simulink model "three_phase_inverter"  (R2021a)
settings: Solver=ode23tb  StartTime=0.0  StopTime=0.5  MaxStep=1e-4  RelTol=1e-3
values from neighbouring files (symbols this model uses):
  Ac = 1    [Inverter_parameters.m]
  Ar = ma*Ac    (= 0.5)    [Inverter_parameters.m]
  Cf = 0.05*Cb    (= 1.42154514158e-05)    [LCL_design.m]
  fc1 = mf1*f    (= 1000)    [Inverter_parameters.m]
  fr = 2*pi*f    (= 314.159265359)    [Inverter_parameters.m]
  L = X/(2*pi*f)    (= 0.0999493042617)    [Inverter_parameters.m]
  L1 = Vdc/(6*Fsw*delta_Imax)    [LCL_design.m]
  L2 = 0.6*L1    [LCL_design.m]
  R = 100    [Inverter_parameters.m]
  Rf = 1/(3*Cf*wres)    [LCL_design.m]
  Vin = 780    [Inverter_parameters.m]
libraries: spsIGBTDiodeLib x6, spsRMSLib x6, spsThreePhaseSeriesRLCBranchLib x4, spsThreePhaseVIMeasurementLib x2, spsCurrentMeasurementLib x1, spsGroundLib x1, spsDCVoltageSourceLib x1, simulink x1, spspowerguiLib x1
settings Model: Creator=HossamAladdin  LastModifiedBy=HossamAladdin
settings DataIOCC: ReturnWorkspaceOutputs=off

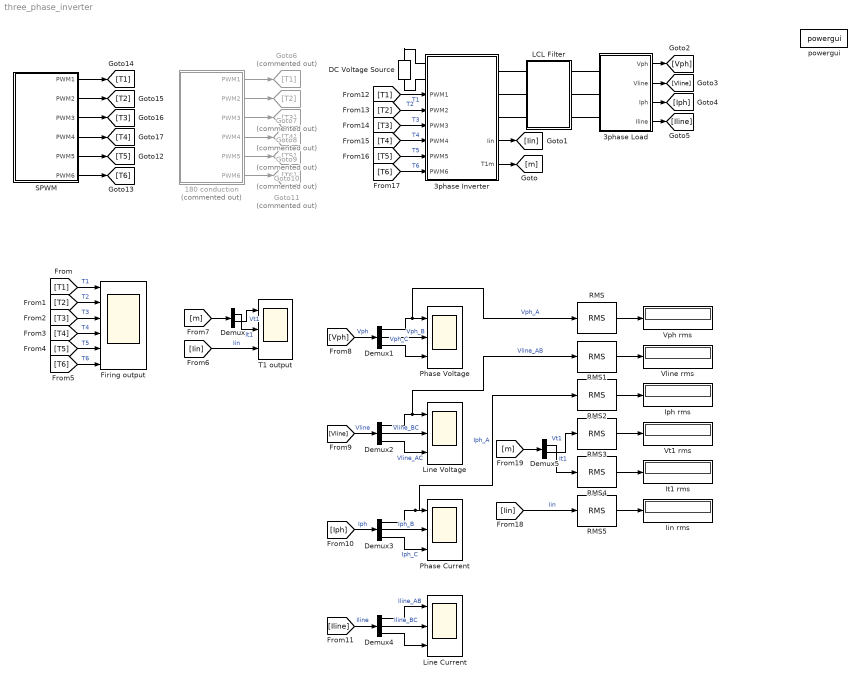
== system three_phase_inverter ==
  180 conduction : Subsystem  Commented=on
  3phase Inverter : Subsystem
      settings: PortSchema="{\"entries\":[{\"content\":{\"sides\":[{\"content\":{\"connectorIds\":[\"LConn1\",\"LConn2\",\"In1\",\"In2\",\"In3\",\"In4\",\"In5\",\"In6\"]},\"type\":\"ConnectorPlacement.EquallySpacedRectSide\",\"uuid\":\"d07aecf3-188f-425b-a441-0ff53fdce9b7\"},{\"content\":{\"connectorIds\":[\"RConn1\",\"RConn2\",\"RConn3\",\"Out1\",\"Out2\"],\"side\":\"RIGHT\"},\"type\":\"ConnectorPlacement.EquallySpacedRectSide\",\"uuid\":\"cba8ab7f-84b3-4f09-b5c1-8f8cbc780d5b\"},{\"content\":{\"connectorIds\":[],\"side\":\"TOP\"},\"type\":\"ConnectorPlacement.EquallySpacedRectSide\",\"uuid\":\"7fc08851-147a-460f-9c9e-af6a73bd199d\"}]},\"type\":\"ConnectorPlacement.EquallySpacedConnector\",\"uuid\":\"b80a74c3-b878-4e7f-834a-08d1a7e19c1c\"}],\"packageUris\":[\"http://schema.mathworks.com/mf0/Connector/R2020b\"],\"version\":\"1.0\"}"
  3phase Load : Subsystem
  DC Voltage Source : spsDCVoltageSourceLib/DC Voltage Source  Amplitude=Vin  Measurements=None
  Demux : Demux  Outputs=2
  Demux{1..4} (4 alike) : Demux  Outputs=3
  Demux5 : Demux  Outputs=2
  Firing output : Scope  NumInputPorts=6
  Goto10 : Goto  Commented=on  GotoTag=T5
  Goto11 : Goto  Commented=on  GotoTag=T6
  Goto6 : Goto  Commented=on  GotoTag=T1
  Goto7 : Goto  Commented=on  GotoTag=T2
  Goto8 : Goto  Commented=on  GotoTag=T3
  Goto9 : Goto  Commented=on  GotoTag=T4
  Iin rms : Display
  Iph rms : Display
  It1 rms : Display
  LCL Filter : Subsystem
  Line Current : Scope  NumInputPorts=3
  Line Voltage : Scope  NumInputPorts=3
  Phase Current : Scope  NumInputPorts=3
  Phase Voltage : Scope  NumInputPorts=3
  RMS{,1..5} (6 alike) : spsRMSLib/RMS  TrueRMS=on  Freq=50  RMSInit=0  Ts=0
  SPWM : Subsystem
  T1 output : Scope  NumInputPorts=3
  Vline rms : Display
  Vph rms : Display
  Vt1 rms : Display
  powergui : spspowerguiLib/powergui  Priority=1  SimulationMode=Discrete  SampleTime=1e-6  frequency=60  Iterations=50  frequencyindice=0  Pbase=100e6  ErrMax=1e-4  UnitsV=kV  UnitsW=MW  buscounter=0  FunctionMessages=off  echomessages=off  EnableUseOfTLC=off  CurrentSourceSwitches=off  DisableSnubberDevices=off  DisableRonSwitches=off  DisableVfSwitches=off  DisplayEquations=off  AutomaticDiscreteSolvers=off  SolverType=Tustin/Backward Euler (TBE)  Interpol=off  ExternalGateDelay=off  methode=off  Ts=100  x0status=blocks  SPID=on  SwTol=0  HookPort=off  NonlinearTolerance=1e-4  nMaxIteration=100  ContinueOnMaxIteration=off  RestoreLinks=warning  ResistiveCurrentMeasurement=off  Frange=[0:2:500]  Ylog=off  Xlog=on  ShowGrid=off  save=off  variable=ZData  structure=0  ZoomFFT=off  StartTime=0.0  cycles=1  DisplayStyle=1  fundamental=60  FreqAxis=off  MaxFrequency=1000  frequencyindicesteady=1  RmsSteady=1  display=off
  wires:
  180 conduction/6(PWM6) -> Goto11/1
  180 conduction/3(PWM3) -> Goto8/1
  180 conduction/1(PWM1) -> Goto6/1
  180 conduction/5(PWM5) -> Goto10/1
  180 conduction/2(PWM2) -> Goto7/1
  180 conduction/4(PWM4) -> Goto9/1
  3phase Inverter/2(T1m) -> [m]
  3phase Inverter/1(Iin) -> [Iin]
  [T1] -> Firing output/1  "T1"
  [T2] -> Firing output/2  "T2"
  [T3] -> Firing output/3  "T3"
  [T4] -> Firing output/4  "T4"
  [T5] -> Firing output/5  "T5"
  [T6] -> Firing output/6  "T6"
  [Iin] -> T1 output/3  "Iin"
  [m] -> Demux/1
  Demux/1 -> T1 output/2  "It1"
  Demux/2 -> T1 output/1  "Vt1"
  3phase Load/1(Vph) -> [Vph]
  3phase Load/2(Vline) -> [Vline]
  3phase Load/3(Iph) -> [Iph]
  3phase Load/4(Iline) -> [Iline]
  [Vph] -> Demux1/1  "Vph"
  [Vline] -> Demux2/1  "Vline"
  [Iph] -> Demux3/1  "Iph"
  [Iline] -> Demux4/1  "Iline"
  [T1] -> 3phase Inverter/1(PWM1)  "T1"
  [T6] -> 3phase Inverter/6(PWM6)  "T6"
  [T5] -> 3phase Inverter/5(PWM5)  "T5"
  [T4] -> 3phase Inverter/4(PWM4)  "T4"
  [T3] -> 3phase Inverter/3(PWM3)  "T3"
  [T2] -> 3phase Inverter/2(PWM2)  "T2"
  SPWM/4(PWM4) -> [T4]
  SPWM/2(PWM2) -> [T2]
  SPWM/5(PWM5) -> [T5]
  SPWM/1(PWM1) -> [T1]
  SPWM/3(PWM3) -> [T3]
  SPWM/6(PWM6) -> [T6]
  Demux1/1 -> RMS/1, Phase Voltage/1  "Vph_A"
  Demux1/2 -> Phase Voltage/2  "Vph_B"
  Demux1/3 -> Phase Voltage/3  "Vph_C"
  Demux2/1 -> RMS1/1, Line Voltage/1  "Vline_AB"
  Demux2/2 -> Line Voltage/2  "Vline_BC"
  Demux2/3 -> Line Voltage/3  "Vline_AC"
  Demux4/1 -> Line Current/1  "Iline_AB"
  Demux4/2 -> Line Current/2  "Iline_BC"
  Demux4/3 -> Line Current/3
  Demux3/1 -> RMS2/1, Phase Current/1  "Iph_A"
  Demux3/2 -> Phase Current/2  "Iph_B"
  Demux3/3 -> Phase Current/3  "Iph_C"
  RMS2/1 -> Iph rms/1
  RMS1/1 -> Vline rms/1
  RMS/1 -> Vph rms/1
  RMS4/1 -> It1 rms/1
  RMS3/1 -> Vt1 rms/1
  Demux5/2 -> RMS3/1  "Vt1"
  Demux5/1 -> RMS4/1  "It1"
  [m] -> Demux5/1
  [Iin] -> RMS5/1  "Iin"
  RMS5/1 -> Iin rms/1
  connections:
  DC Voltage Source/RConn1 -- 3phase Inverter/LConn1
  DC Voltage Source/LConn1 -- 3phase Inverter/LConn2
  LCL Filter/RConn1 -- 3phase Load/LConn1
  LCL Filter/RConn2 -- 3phase Load/LConn2
  LCL Filter/RConn3 -- 3phase Load/LConn3
  LCL Filter/LConn3 -- 3phase Inverter/RConn3
  LCL Filter/LConn1 -- 3phase Inverter/RConn1
  LCL Filter/LConn2 -- 3phase Inverter/RConn2

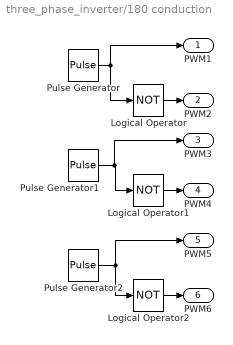
== system three_phase_inverter/180 conduction ==
  Logical Operator : Logic  Operator=NOT  AllPortsSameDT=off  OutDataTypeStr=boolean
  Logical Operator1 : Logic  Operator=NOT  AllPortsSameDT=off  OutDataTypeStr=boolean
  Logical Operator2 : Logic  Operator=NOT  AllPortsSameDT=off  OutDataTypeStr=boolean
  Pulse Generator : DiscretePulseGenerator  PulseType=Time based  Period=t  PulseWidth=50
  Pulse Generator1 : DiscretePulseGenerator  PulseType=Time based  Period=t  PulseWidth=50  PhaseDelay=(120*t)/360
  Pulse Generator2 : DiscretePulseGenerator  PulseType=Time based  Period=t  PulseWidth=50  PhaseDelay=(240*t)/360
  PWM1 : Outport
  PWM2 : Outport  Port=2
  PWM3 : Outport  Port=3
  PWM4 : Outport  Port=4
  PWM5 : Outport  Port=5
  PWM6 : Outport  Port=6
  wires:
  Logical Operator2/1 -> PWM6/1
  Logical Operator1/1 -> PWM4/1
  Pulse Generator/1 -> PWM1/1, Logical Operator/1
  Pulse Generator2/1 -> PWM5/1, Logical Operator2/1
  Pulse Generator1/1 -> PWM3/1, Logical Operator1/1
  Logical Operator/1 -> PWM2/1

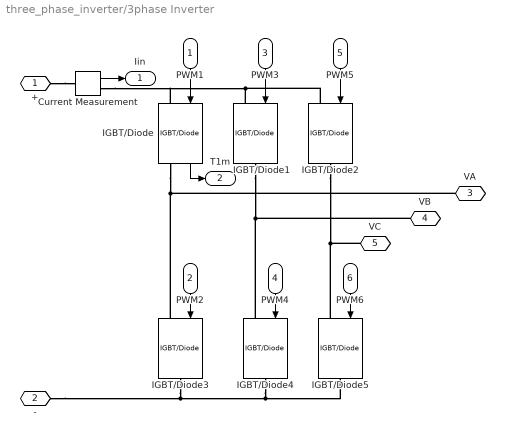
== system three_phase_inverter/3phase Inverter ==
  PWM1 : Inport
  PWM2 : Inport  Port=2
  PWM3 : Inport  Port=3
  PWM4 : Inport  Port=4
  PWM5 : Inport  Port=5
  PWM6 : Inport  Port=6
  Current Measurement : spsCurrentMeasurementLib/Current Measurement  PhasorSimulation=off  OutputType=Complex  PSBequivalent=0
  IGBT/Diode : spsIGBTDiodeLib/IGBT//Diode  Ron=1e-3  Rs=1e5  Cs=inf  Measurements=on
  IGBT/Diode{1..5} (5 alike) : spsIGBTDiodeLib/IGBT//Diode  Ron=1e-3  Rs=1e5  Cs=inf  Measurements=off
  + : PMIOPort  Side=Left
  - : PMIOPort  Port=2  Side=Left
  VA : PMIOPort  Port=3  Side=Right
  VB : PMIOPort  Port=4  Side=Right
  VC : PMIOPort  Port=5  Side=Right
  Iin : Outport
  T1m : Outport  Port=2
  wires:
  PWM1/1 -> IGBT/Diode/1
  PWM3/1 -> IGBT/Diode1/1
  PWM6/1 -> IGBT/Diode5/1
  PWM4/1 -> IGBT/Diode4/1
  PWM5/1 -> IGBT/Diode2/1
  PWM2/1 -> IGBT/Diode3/1
  IGBT/Diode/1 -> T1m/1
  Current Measurement/1 -> Iin/1
  connections:
  IGBT/Diode3/RConn1 -- IGBT/Diode5/RConn1 -- IGBT/Diode4/RConn1 -- -/RConn1
  IGBT/Diode2/LConn1 -- Current Measurement/RConn1 -- IGBT/Diode/LConn1 -- IGBT/Diode1/LConn1
  IGBT/Diode1/RConn1 -- VB/RConn1 -- IGBT/Diode4/LConn1
  IGBT/Diode2/RConn1 -- VC/RConn1 -- IGBT/Diode5/LConn1
  VA/RConn1 -- IGBT/Diode/RConn1 -- IGBT/Diode3/LConn1
  +/RConn1 -- Current Measurement/LConn1

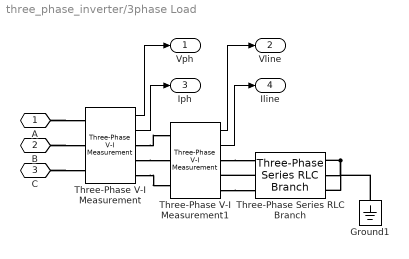
== system three_phase_inverter/3phase Load ==
  Ground1 : spsGroundLib/Ground  LConnTagsString=a
  Three-Phase Series RLC Branch : spsThreePhaseSeriesRLCBranchLib/Three-Phase Series RLC Branch  LConnTagsString=A|B|C  RConnTagsString=A|B|C  BranchType=RL  Resistance=R  Inductance=L  Capacitance=1e-6  Measurements=None
  Three-Phase V-I Measurement : spsThreePhaseVIMeasurementLib/Three-Phase V-I Measurement  VoltageMeasurement=phase-to-ground  SetLabelV=off  LabelV=Vabc  Vpu=off  VpuLL=off  CurrentMeasurement=yes  SetLabelI=off  LabelI=Iabc  Ipu=off  Pbase=100e6  Vbase=500e3  OutputType=Complex  PhasorSimulation=off  PSBequivalent=0
  Three-Phase V-I Measurement1 : spsThreePhaseVIMeasurementLib/Three-Phase V-I Measurement  VoltageMeasurement=phase-to-phase  SetLabelV=off  LabelV=Vabc  Vpu=off  VpuLL=off  CurrentMeasurement=yes  SetLabelI=off  LabelI=Iabc  Ipu=off  Pbase=100e6  Vbase=500e3  OutputType=Complex  PhasorSimulation=off  PSBequivalent=0
  A : PMIOPort  Side=Left
  B : PMIOPort  Port=2  Side=Left
  C : PMIOPort  Port=3  Side=Left
  Vph : Outport
  Vline : Outport  Port=2
  Iph : Outport  Port=3
  Iline : Outport  Port=4
  wires:
  Three-Phase V-I Measurement/1 -> Vph/1
  Three-Phase V-I Measurement1/1 -> Vline/1
  Three-Phase V-I Measurement/2 -> Iph/1
  Three-Phase V-I Measurement1/2 -> Iline/1
  connections:
  Three-Phase V-I Measurement1/RConn1 -- Three-Phase Series RLC Branch/LConn1
  Three-Phase V-I Measurement1/RConn3 -- Three-Phase Series RLC Branch/LConn3
  Three-Phase Series RLC Branch/LConn2 -- Three-Phase V-I Measurement1/RConn2
  Three-Phase Series RLC Branch/RConn1 -- Three-Phase Series RLC Branch/RConn2 -- Ground1/LConn1 -- Three-Phase Series RLC Branch/RConn3
  Three-Phase V-I Measurement/RConn1 -- Three-Phase V-I Measurement1/LConn1
  Three-Phase V-I Measurement/RConn2 -- Three-Phase V-I Measurement1/LConn2
  Three-Phase V-I Measurement/RConn3 -- Three-Phase V-I Measurement1/LConn3
  A/RConn1 -- Three-Phase V-I Measurement/LConn1
  B/RConn1 -- Three-Phase V-I Measurement/LConn2
  C/RConn1 -- Three-Phase V-I Measurement/LConn3

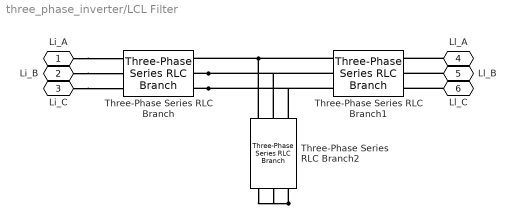
== system three_phase_inverter/LCL Filter ==
  Three-Phase Series RLC Branch : spsThreePhaseSeriesRLCBranchLib/Three-Phase Series RLC Branch  LConnTagsString=A|B|C  RConnTagsString=A|B|C  BranchType=L  Resistance=R  Inductance=L1  Capacitance=1e-6  Measurements=None
  Three-Phase Series RLC Branch1 : spsThreePhaseSeriesRLCBranchLib/Three-Phase Series RLC Branch  LConnTagsString=A|B|C  RConnTagsString=A|B|C  BranchType=L  Resistance=R  Inductance=L2  Capacitance=1e-6  Measurements=None
  Three-Phase Series RLC Branch2 : spsThreePhaseSeriesRLCBranchLib/Three-Phase Series RLC Branch  LConnTagsString=A|B|C  RConnTagsString=A|B|C  BranchType=RC  Resistance=Rf  Inductance=L  Capacitance=Cf  Measurements=None
  Li_A : PMIOPort  Side=Left
  Li_B : PMIOPort  Port=2  Side=Left
  Li_C : PMIOPort  Port=3  Side=Left
  Ll_A : PMIOPort  Port=4  Side=Right
  Ll_B : PMIOPort  Port=5  Side=Right
  Ll_C : PMIOPort  Port=6  Side=Right
  connections:
  Li_A/RConn1 -- Three-Phase Series RLC Branch/LConn1
  Li_B/RConn1 -- Three-Phase Series RLC Branch/LConn2
  Li_C/RConn1 -- Three-Phase Series RLC Branch/LConn3
  Three-Phase Series RLC Branch1/LConn1 -- Three-Phase Series RLC Branch2/LConn1 -- Three-Phase Series RLC Branch/RConn1
  Three-Phase Series RLC Branch/RConn3 -- Three-Phase Series RLC Branch2/LConn3 -- Three-Phase Series RLC Branch1/LConn3
  Three-Phase Series RLC Branch/RConn2 -- Three-Phase Series RLC Branch2/LConn2 -- Three-Phase Series RLC Branch1/LConn2
  Three-Phase Series RLC Branch2/RConn3 -- Three-Phase Series RLC Branch2/RConn1 -- Three-Phase Series RLC Branch2/RConn2
  Ll_A/RConn1 -- Three-Phase Series RLC Branch1/RConn1
  Ll_B/RConn1 -- Three-Phase Series RLC Branch1/RConn2
  Ll_C/RConn1 -- Three-Phase Series RLC Branch1/RConn3

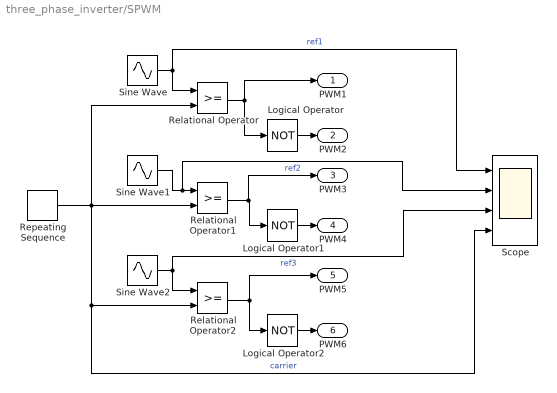
== system three_phase_inverter/SPWM ==
  Logical Operator : Logic  Operator=NOT  AllPortsSameDT=off  OutDataTypeStr=boolean
  Logical Operator1 : Logic  Operator=NOT  AllPortsSameDT=off  OutDataTypeStr=boolean
  Logical Operator2 : Logic  Operator=NOT  AllPortsSameDT=off  OutDataTypeStr=boolean
  Relational Operator : RelationalOperator  OutDataTypeStr=boolean  RndMeth=Simplest
  Relational Operator1 : RelationalOperator  OutDataTypeStr=boolean  RndMeth=Simplest
  Relational Operator2 : RelationalOperator  OutDataTypeStr=boolean  RndMeth=Simplest
  Repeating Sequence : simulink/Sources/Repeating Sequence  rep_seq_t=[0 (1/fc1)/4 (1/fc1)/2 (3/fc1)/4 (1/fc1)]  rep_seq_y=[0 Ac 0 -Ac 0]
  Scope : Scope  NumInputPorts=4
  Sine Wave : Sin  Amplitude=Ar  Frequency=fr  SampleTime=0
  Sine Wave1 : Sin  Amplitude=Ar  Frequency=fr  Phase=(2*pi)/3  SampleTime=0
  Sine Wave2 : Sin  Amplitude=Ar  Frequency=fr  Phase=(4*pi)/3  SampleTime=0
  PWM1 : Outport
  PWM2 : Outport  Port=2
  PWM3 : Outport  Port=3
  PWM4 : Outport  Port=4
  PWM5 : Outport  Port=5
  PWM6 : Outport  Port=6
  wires:
  Logical Operator/1 -> PWM2/1
  Relational Operator1/1 -> Logical Operator1/1, PWM3/1
  Relational Operator2/1 -> Logical Operator2/1, PWM5/1
  Relational Operator/1 -> Logical Operator/1, PWM1/1
  Logical Operator1/1 -> PWM4/1
  Logical Operator2/1 -> PWM6/1
  Sine Wave/1 -> Relational Operator/1, Scope/1  "ref1"
  Sine Wave1/1 -> Scope/2, Relational Operator1/1  "ref2"
  Repeating Sequence/1 -> Relational Operator/2, Relational Operator1/2, Relational Operator2/2, Scope/4  "carrier"
  Sine Wave2/1 -> Relational Operator2/1, Scope/3  "ref3"
